simulink model "WEEK1_QN5"  (R2020b)
settings: Solver=VariableStepAuto  StartTime=0.0  StopTime=10.0  RelTol=1e-3
model workspace (MAT data in the model file):
  C = 1e-05
  R = 10
settings Model: Creator=dell  LastModifiedBy=dell

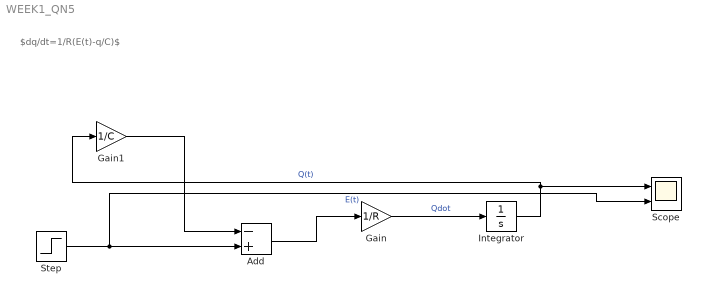
== system WEEK1_QN5 ==
  note: $dq/dt=1/R(E(t)-q/C)$
  Add : Sum  Inputs=-+
  Gain : Gain  Gain=1/R
  Gain1 : Gain  Gain=1/C
  Integrator : Integrator  InitialCondition=9
  Scope : Scope  NumInputPorts=2
  Step : Step  SampleTime=0
  wires:
  Integrator/1 -> Scope/1, Gain1/1  "Q(t)"
  Step/1 -> Scope/2, Add/2  "E(t)"
  Gain/1 -> Integrator/1  "Qdot"
  Gain1/1 -> Add/1
  Add/1 -> Gain/1
